simulink model "impedance_control"  (R2020b)
settings: Solver=FixedStepAuto  StartTime=0.0  StopTime=10  FixedStep=Ts  RelTol=1e-3
undefined symbols (not defined in the file): dqi, invMd, K, KD, KP, Md, myRobot, qi, xf, xi, xr
settings Model: Creator=simon  LastModifiedBy=SimoneCremasco
settings SolverCC: ZeroCrossControl=DisableAll

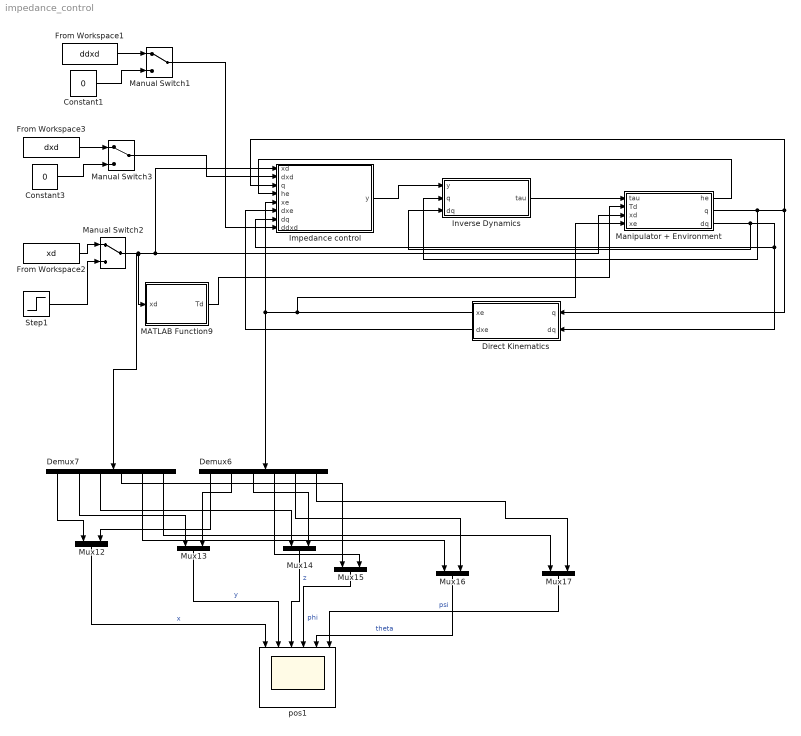
== system impedance_control ==
  Constant1 : Constant  Value=0
  Constant3 : Constant  Value=0
  Demux6 : Demux  Outputs=6
  Demux7 : Demux  Outputs=6
  Direct Kinematics : Subsystem
  From Workspace1 : FromWorkspace  VariableName=ddxd
  From Workspace2 : FromWorkspace  VariableName=xd
  From Workspace3 : FromWorkspace  VariableName=dxd
  Impedance control : Subsystem
  Inverse Dynamics : Subsystem
  MATLAB Function9 : MATLAB Function  TreatAsAtomicUnit=on
  Manipulator + Environment : Subsystem
  Manual Switch1 : ManualSwitch
  Manual Switch2 : ManualSwitch
  Manual Switch3 : ManualSwitch
  Mux{12..17} (6 alike) : Mux  Inputs=2
  Step1 : Step  Before=xi  After=xf  SampleTime=0
  pos1 : Scope  NumInputPorts=6
  wires:
  Direct Kinematics/2(dxe) -> Impedance control/6(dxe)
  Impedance control/1(y) -> Inverse Dynamics/1(y)
  Inverse Dynamics/1(tau) -> Manipulator + Environment/1(tau)
  Manipulator + Environment/2(q) -> Inverse Dynamics/2(q), Impedance control/3(q), Direct Kinematics/1(q)
  Manipulator + Environment/3(dq) -> Inverse Dynamics/3(dq), Impedance control/7(dq), Direct Kinematics/2(dq)
  Manipulator + Environment/1(he) -> Impedance control/4(he)
  Step1/1 -> Manual Switch2/2
  From Workspace2/1 -> Manual Switch2/1
  From Workspace3/1 -> Manual Switch3/1
  Constant3/1 -> Manual Switch3/2
  Manual Switch3/1 -> Impedance control/2(dxd)
  MATLAB Function9/1(Td) -> Manipulator + Environment/2(Td)
  Demux7/3 -> Mux14/1
  Direct Kinematics/1(xe) -> Demux6/1, Impedance control/5(xe), Manipulator + Environment/4(xe)
  Mux17/1 -> pos1/6  "psi"
  Demux6/5 -> Mux16/2
  Demux7/6 -> Mux17/1
  Mux16/1 -> pos1/5  "theta"
  Mux15/1 -> pos1/4  "phi"
  Manual Switch2/1 -> Demux7/1, MATLAB Function9/1(xd), Manipulator + Environment/3(xd), Impedance control/1(xd)
  Demux7/4 -> Mux15/1
  Demux7/2 -> Mux13/1
  Demux6/6 -> Mux17/2
  Mux14/1 -> pos1/3  "z"
  Demux7/1 -> Mux12/1
  Demux6/2 -> Mux13/2
  Demux7/5 -> Mux16/1
  Demux6/1 -> Mux12/2
  Demux6/3 -> Mux14/2
  Mux12/1 -> pos1/1  "x"
  Demux6/4 -> Mux15/2
  Mux13/1 -> pos1/2  "y"
  Constant1/1 -> Manual Switch1/2
  From Workspace1/1 -> Manual Switch1/1
  Manual Switch1/1 -> Impedance control/8(ddxd)

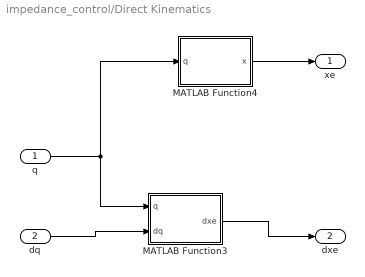
== system impedance_control/Direct Kinematics ==
  q : Inport
  dq : Inport  Port=2
  MATLAB Function3 : MATLAB Function  TreatAsAtomicUnit=on
  MATLAB Function4 : MATLAB Function  TreatAsAtomicUnit=on
  xe : Outport
  dxe : Outport  Port=2
  wires:
  MATLAB Function3/1(dxe) -> dxe/1
  dq/1 -> MATLAB Function3/2(dq)
  q/1 -> MATLAB Function4/1(q), MATLAB Function3/1(q)
  MATLAB Function4/1(x) -> xe/1

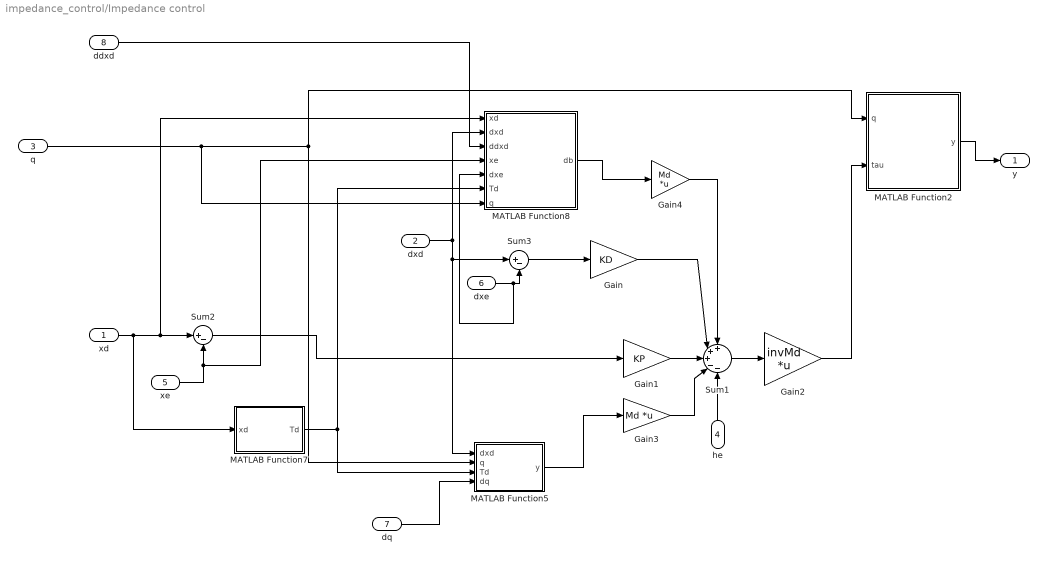
== system impedance_control/Impedance control ==
  xd : Inport
  dxd : Inport  Port=2
  q : Inport  Port=3
  he : Inport  Port=4
  xe : Inport  Port=5
  dxe : Inport  Port=6
  dq : Inport  Port=7
  ddxd : Inport  Port=8
  Gain : Gain  Gain=KD
  Gain1 : Gain  Gain=KP
  Gain2 : Gain  Gain=invMd  Multiplication=Matrix(K*u)
  Gain3 : Gain  Gain=Md  Multiplication=Matrix(K*u)
  Gain4 : Gain  Gain=Md  Multiplication=Matrix(K*u)
  MATLAB Function2 : MATLAB Function  TreatAsAtomicUnit=on
  MATLAB Function5 : MATLAB Function  TreatAsAtomicUnit=on
  MATLAB Function7 : MATLAB Function  TreatAsAtomicUnit=on
  MATLAB Function8 : MATLAB Function  TreatAsAtomicUnit=on
  Sum1 : Sum  Inputs=+++--
  Sum2 : Sum  Inputs=|+-
  Sum3 : Sum  Inputs=|+-
  y : Outport
  wires:
  MATLAB Function7/1(Td) -> MATLAB Function5/3(Td), MATLAB Function8/6(Td)
  MATLAB Function8/1(db) -> Gain4/1
  MATLAB Function5/1(y) -> Gain3/1
  Gain2/1 -> MATLAB Function2/2(tau)
  dxd/1 -> MATLAB Function5/1(dxd), Sum3/1, MATLAB Function8/2(dxd)
  xd/1 -> MATLAB Function8/1(xd), Sum2/1, MATLAB Function7/1(xd)
  Gain3/1 -> Sum1/4
  MATLAB Function2/1(y) -> y/1
  Gain/1 -> Sum1/2
  Sum3/1 -> Gain/1
  Sum1/1 -> Gain2/1
  Gain1/1 -> Sum1/3
  Sum2/1 -> Gain1/1
  Gain4/1 -> Sum1/1
  he/1 -> Sum1/5
  q/1 -> MATLAB Function8/7(q), MATLAB Function5/2(q), MATLAB Function2/1(q)
  xe/1 -> MATLAB Function8/4(xe), Sum2/2
  dxe/1 -> MATLAB Function8/5(dxe), Sum3/2
  dq/1 -> MATLAB Function5/4(dq)
  ddxd/1 -> MATLAB Function8/3(ddxd)

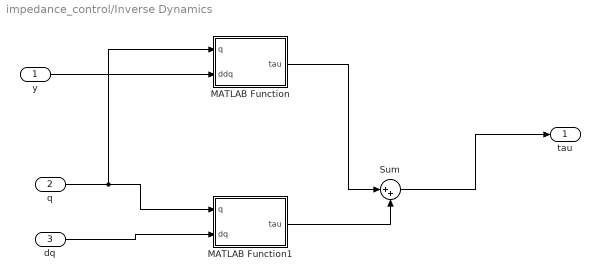
== system impedance_control/Inverse Dynamics ==
  y : Inport
  q : Inport  Port=2
  dq : Inport  Port=3
  MATLAB Function : MATLAB Function  TreatAsAtomicUnit=on
  MATLAB Function1 : MATLAB Function  TreatAsAtomicUnit=on
  Sum : Sum  Inputs=|++
  tau : Outport
  wires:
  MATLAB Function1/1(tau) -> Sum/2
  MATLAB Function/1(tau) -> Sum/1
  y/1 -> MATLAB Function/2(ddq)
  Sum/1 -> tau/1
  dq/1 -> MATLAB Function1/2(dq)
  q/1 -> MATLAB Function/1(q), MATLAB Function1/1(q)

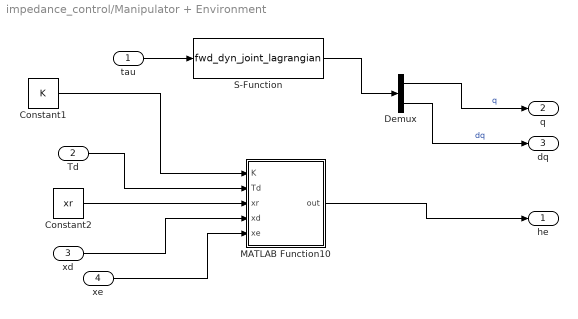
== system impedance_control/Manipulator + Environment ==
  tau : Inport
  Td : Inport  Port=2
  xd : Inport  Port=3
  xe : Inport  Port=4
  Constant1 : Constant  Value=K
  Constant2 : Constant  Value=xr
  Demux : Demux  Outputs=2
  MATLAB Function10 : MATLAB Function  TreatAsAtomicUnit=on
  S-Function : S-Function  FunctionName=fwd_dyn_joint_lagrangian  Parameters=myRobot,qi,dqi  SFunctionDeploymentMode=off  EnableBusSupport=off
  he : Outport
  q : Outport  Port=2
  dq : Outport  Port=3
  wires:
  tau/1 -> S-Function/1
  Constant1/1 -> MATLAB Function10/1(K)
  Constant2/1 -> MATLAB Function10/3(xr)
  Td/1 -> MATLAB Function10/2(Td)
  xd/1 -> MATLAB Function10/4(xd)
  xe/1 -> MATLAB Function10/5(xe)
  S-Function/1 -> Demux/1
  Demux/1 -> q/1  "q"
  Demux/2 -> dq/1  "dq"
  MATLAB Function10/1(out) -> he/1

== matlab function impedance_control/Direct Kinematics/MATLAB Function3 ==
  data: q input; dxe output; dq input
function dxe = Ja(q, dq)

dxe = getJa(q)*dq;

== matlab function impedance_control/Impedance control/MATLAB Function2 ==
  data: q input; y output; tau input
function y = invJa(q, tau)

y = getInvJa(q)*tau;

== matlab function impedance_control/Direct Kinematics/MATLAB Function4 ==
  data: q input; x output
function x = k(q)

x = getK(q);

== matlab function impedance_control/Impedance control/MATLAB Function5 ==
  data: dxd input; q input; Td input; y output; dq input
function y = dJadq(dxd, q, Td,dq)
    y = getDiffJad(dxd,q,Td)*dq;

== matlab function impedance_control/Impedance control/MATLAB Function7 ==
  data: xd input; Td output
function Td = getTd(xd)
Rd = eul2rotm(xd(4:6)','ZYZ');
t = xd(1:3);
Td = [Rd t
    zeros(1,3) 1];

== matlab function impedance_control/Impedance control/MATLAB Function8 ==
  data: xd input; dxd input; ddxd input; xe input; dxe input; db output; Td input; q input
function db = diffB(xd,dxd,ddxd,xe,dxe, Td,q)

db = getDiffImpB(xd,dxd,ddxd,xe,dxe, Td,q);

== matlab function impedance_control/Inverse Dynamics/MATLAB Function ==
  data: q input size=3; tau output; ddq input size=3
function tau = B(q, ddq)

tau = getB(q)*ddq;

== matlab function impedance_control/Inverse Dynamics/MATLAB Function1 ==
  data: q input size=3; tau output; dq input size=3
function tau = n(q, dq)

tau = getN(q, dq);

== matlab function impedance_control/Manipulator + Environment/MATLAB Function10 ==
  data: K input; Td input; out output size=6; xr input; xd input; xe input size=6
function out = hde(K,Td, xr, xd, xe)
%consider the interaction only in z direction
if xe(3) < xr(3)
    dxrd = xd-xr;
    dxed = xd-xe;
    dxre = dxrd-dxed;
    he = K*dxre;
else
    he = zeros(6,1);
end

out = he;

== matlab function impedance_control/MATLAB Function9 ==
  data: xd input; Td output
function Td = getTd(xd)
Rd = eul2rotm(xd(4:6)','ZYZ');
t = xd(1:3);
Td = [Rd t
    zeros(1,3) 1];
